simulink model "BWQWFPIDa"  (Simulink 8.3)
settings: Solver=ode45  SolverMode=SingleTasking  StartTime=0.0  StopTime=1000  FixedStep=20  RelTol=1e-3
settings Model: Creator=Zhu Supeng  LastModifiedBy=Zhu Supeng
settings DataIOCC: SignalLoggingName=sigsOut
settings DebuggingCC: SaveWithParameterizedLinksMsg=none  SignalResolutionControl=TryResolveAllWithWarning  SolverPrmCheckMsg=none  MultiTaskDSMMsg=warning  MultiTaskCondExecSysMsg=none  StateNameClashWarn=none
settings HardwareCC: TargetUnknown=on
settings RTWCC: IncludeERTFirstTime=on

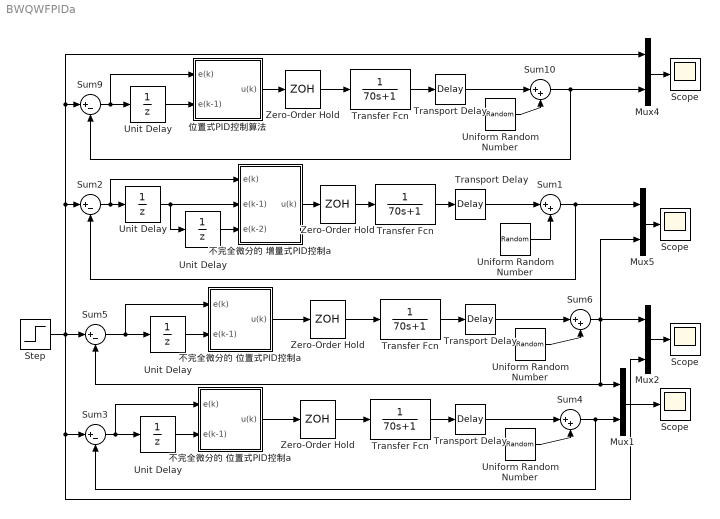
== system BWQWFPIDa ==
  "  Scope " : Scope
      settings: YMin=-3.5  YMax=1  SaveName=ScopeData3  MaxDataPoints=500000
  "  Transfer Fcn  " : TransferFcn  Denominator=[70 1]
  "  Transport Delay " : TransportDelay  DelayTime=80
  "  Unit Delay  " : UnitDelay  SampleTime=20
  " Scope " : Scope
      settings: YMin=-3.5  YMax=1  SaveName=BWQWFPIDary  MaxDataPoints=500000
  " Transfer Fcn " : TransferFcn  Denominator=[70 1]
  " Transport Delay " : TransportDelay  DelayTime=80
  " Unit Delay " : UnitDelay  SampleTime=20
  " Zero-Order Hold   " : ZeroOrderHold  SampleTime=20
  " 不完全微分的 位置式PID控制a " : Subsystem
  Mux1 : Mux  Inputs=2
  Mux2 : Mux  Inputs=3
  Mux4 : Mux  Inputs=2
  Mux5 : Mux  Inputs=2
  Scope : Scope
      settings: YMin=-3.5  YMax=1  MaxDataPoints=500000
  "Scope " : Scope
      settings: YMin=-3.5  YMax=1  MaxDataPoints=500000
  Step : Step  Time=0  SampleTime=0
  Sum{1,4,6,10} (4 alike) : Sum  Inputs=|++  SaturateOnIntegerOverflow=on
  Sum{2..3,5,9} (4 alike) : Sum  Inputs=|+-  SaturateOnIntegerOverflow=on
  Transfer Fcn : TransferFcn  Denominator=[70 1]
  "Transfer Fcn " : TransferFcn  Denominator=[70 1]
  Transport Delay : TransportDelay  DelayTime=80
  "Transport Delay " : TransportDelay  DelayTime=80
  Uniform Random Number : UniformRandomNumber  Minimum=-0.01  Maximum=0.01  SampleTime=20
  "Uniform Random Number " : UniformRandomNumber  Minimum=-0.01  Maximum=0.01  SampleTime=20
  "Uniform Random Number  " : UniformRandomNumber  Minimum=-0.01  Maximum=0.01  SampleTime=20
  "Uniform Random Number    " : UniformRandomNumber  Minimum=-0.01  Maximum=0.01  SampleTime=20
  Unit Delay : UnitDelay  SampleTime=20
  "Unit Delay " : UnitDelay  SampleTime=20
  "Unit Delay  " : UnitDelay  SampleTime=20
  Zero-Order Hold : ZeroOrderHold  SampleTime=20
  "Zero-Order Hold " : ZeroOrderHold  SampleTime=20
  "Zero-Order Hold  " : ZeroOrderHold  SampleTime=20
  不完全微分的 位置式PID控制a : Subsystem
  不完全微分的 增量式PID控制a : Subsystem
  "位置式PID控制算法 " : Subsystem
  wires:
  Step/1 -> Sum9/1, Mux4/1, Sum2/1, Sum5/1, Sum3/1, Mux2/3
  Transfer Fcn/1 -> Transport Delay/1
  "位置式PID控制算法 "/1(u(k)) -> Zero-Order Hold/1
  Unit Delay/1 -> "位置式PID控制算法 "/2(e(k-1))
  Sum9/1 -> Unit Delay/1, "位置式PID控制算法 "/1(e(k))
  Zero-Order Hold/1 -> Transfer Fcn/1
  Uniform Random Number/1 -> Sum10/2
  Transport Delay/1 -> Sum10/1
  Sum10/1 -> Sum9/2, Mux4/2
  Mux4/1 -> Scope/1
  "Transfer Fcn "/1 -> "Transport Delay "/1
  不完全微分的 增量式PID控制a/1(u(k)) -> "Zero-Order Hold "/1
  Sum2/1 -> "Unit Delay "/1, 不完全微分的 增量式PID控制a/1(e(k))
  Mux5/1 -> "Scope "/1
  "Transport Delay "/1 -> Sum1/1
  Sum1/1 -> Mux5/1, Sum2/2
  "Zero-Order Hold "/1 -> "Transfer Fcn "/1
  "Unit Delay "/1 -> "Unit Delay  "/1, 不完全微分的 增量式PID控制a/2(e(k-1))
  "Unit Delay  "/1 -> 不完全微分的 增量式PID控制a/3(e(k-2))
  " Transfer Fcn "/1 -> " Transport Delay "/1
  不完全微分的 位置式PID控制a/1(u(k)) -> "Zero-Order Hold  "/1
  " Unit Delay "/1 -> 不完全微分的 位置式PID控制a/2(e(k-1))
  Sum5/1 -> " Unit Delay "/1, 不完全微分的 位置式PID控制a/1(e(k))
  Mux2/1 -> " Scope "/1
  "Uniform Random Number  "/1 -> Sum6/2
  Sum6/1 -> Mux2/1, Mux5/2, Sum5/2, Mux1/1
  " Transport Delay "/1 -> Sum6/1
  "Zero-Order Hold  "/1 -> " Transfer Fcn "/1
  "Uniform Random Number "/1 -> Sum1/2
  "  Transfer Fcn  "/1 -> "  Transport Delay "/1
  " 不完全微分的 位置式PID控制a "/1(u(k)) -> " Zero-Order Hold   "/1
  "  Unit Delay  "/1 -> " 不完全微分的 位置式PID控制a "/2(e(k-1))
  Sum3/1 -> " 不完全微分的 位置式PID控制a "/1(e(k)), "  Unit Delay  "/1
  "Uniform Random Number    "/1 -> Sum4/2
  "  Transport Delay "/1 -> Sum4/1
  " Zero-Order Hold   "/1 -> "  Transfer Fcn  "/1
  Mux1/1 -> "  Scope "/1
  Sum4/1 -> Mux1/2, Sum3/2

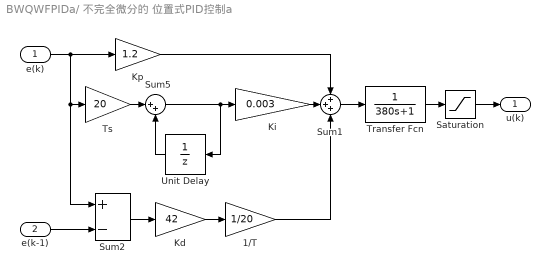
== system BWQWFPIDa/ 不完全微分的 位置式PID控制a  ==
  e(k) : Inport
  e(k-1) : Inport  Port=2
  1/T : Gain  Gain=1/20  SaturateOnIntegerOverflow=on  OutDataTypeStr=Inherit: Same as input  ParamDataTypeStr=Inherit: Same as input
  Kd : Gain  Gain=42  SaturateOnIntegerOverflow=on  OutDataTypeStr=Inherit: Same as input  ParamDataTypeStr=Inherit: Same as input
  Ki : Gain  Gain=0.003  SaturateOnIntegerOverflow=on  OutDataTypeStr=Inherit: Same as input  ParamDataTypeStr=Inherit: Same as input
  Kp : Gain  Gain=1.2  SaturateOnIntegerOverflow=on  OutDataTypeStr=Inherit: Same as input  ParamDataTypeStr=Inherit: Same as input
  Saturation : Saturate  UpperLimit=10  LowerLimit=-10
  Sum1 : Sum  Inputs=+++  SaturateOnIntegerOverflow=on
  Sum2 : Sum  Inputs=+-  SaturateOnIntegerOverflow=on
  Sum5 : Sum  Inputs=|++  SaturateOnIntegerOverflow=on
  Transfer Fcn : TransferFcn  Denominator=[380 1]
  Ts : Gain  Gain=20  SaturateOnIntegerOverflow=on  OutDataTypeStr=Inherit: Same as input  ParamDataTypeStr=Inherit: Same as input
  Unit Delay : UnitDelay  SampleTime=20
  u(k) : Outport
  wires:
  Ki/1 -> Sum1/2
  1/T/1 -> Sum1/3
  Sum2/1 -> Kd/1
  e(k)/1 -> Kp/1, Ts/1, Sum2/1
  Kp/1 -> Sum1/1
  e(k-1)/1 -> Sum2/2
  Kd/1 -> 1/T/1
  Ts/1 -> Sum5/1
  Sum5/1 -> Unit Delay/1, Ki/1
  Unit Delay/1 -> Sum5/2
  Sum1/1 -> Transfer Fcn/1
  Saturation/1 -> u(k)/1
  Transfer Fcn/1 -> Saturation/1

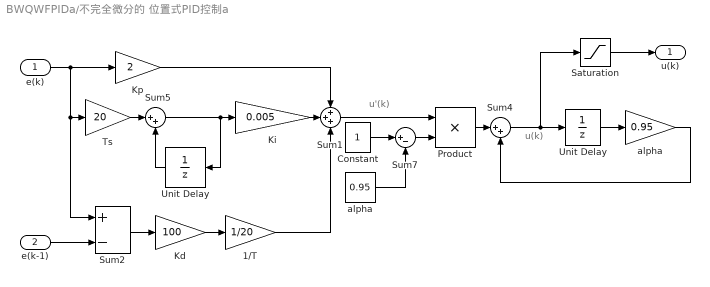
== system BWQWFPIDa/不完全微分的 位置式PID控制a ==
  note: u'(k)
  note: u(k)
  e(k) : Inport
  e(k-1) : Inport  Port=2
  1/T : Gain  Gain=1/20  SaturateOnIntegerOverflow=on  OutDataTypeStr=Inherit: Same as input  ParamDataTypeStr=Inherit: Same as input
  Constant : Constant
  Kd : Gain  Gain=100  SaturateOnIntegerOverflow=on  OutDataTypeStr=Inherit: Same as input  ParamDataTypeStr=Inherit: Same as input
  Ki : Gain  Gain=0.005  SaturateOnIntegerOverflow=on  OutDataTypeStr=Inherit: Same as input  ParamDataTypeStr=Inherit: Same as input
  Kp : Gain  Gain=2  SaturateOnIntegerOverflow=on  OutDataTypeStr=Inherit: Same as input  ParamDataTypeStr=Inherit: Same as input
  Product : Product  SaturateOnIntegerOverflow=on  OutDataTypeStr=Inherit: Same as first input
  Saturation : Saturate  UpperLimit=10  LowerLimit=-10
  Sum1 : Sum  Inputs=+++  SaturateOnIntegerOverflow=on
  Sum2 : Sum  Inputs=+-  SaturateOnIntegerOverflow=on
  Sum4 : Sum  Inputs=|++  SaturateOnIntegerOverflow=on
  Sum5 : Sum  Inputs=|++  SaturateOnIntegerOverflow=on
  Sum7 : Sum  Inputs=|+-  SaturateOnIntegerOverflow=on
  Ts : Gain  Gain=20  SaturateOnIntegerOverflow=on  OutDataTypeStr=Inherit: Same as input  ParamDataTypeStr=Inherit: Same as input
  Unit Delay : UnitDelay  SampleTime=20
  "Unit Delay " : UnitDelay  SampleTime=20
  alpha : Constant  Value=0.95
  "alpha " : Gain  Gain=0.95  SaturateOnIntegerOverflow=on  OutDataTypeStr=Inherit: Same as input  ParamDataTypeStr=Inherit: Same as input
  u(k) : Outport
  wires:
  "alpha "/1 -> Sum4/2
  "Unit Delay "/1 -> "alpha "/1
  Sum4/1 -> Saturation/1, "Unit Delay "/1
  Unit Delay/1 -> Sum5/2
  Sum5/1 -> Ki/1, Unit Delay/1
  Ts/1 -> Sum5/1
  Kd/1 -> 1/T/1
  e(k-1)/1 -> Sum2/2
  Saturation/1 -> u(k)/1
  Kp/1 -> Sum1/1
  e(k)/1 -> Sum2/1, Ts/1, Kp/1
  alpha/1 -> Sum7/2
  Constant/1 -> Sum7/1
  Sum2/1 -> Kd/1
  Product/1 -> Sum4/1
  Sum1/1 -> Product/1
  1/T/1 -> Sum1/3
  Ki/1 -> Sum1/2
  Sum7/1 -> Product/2

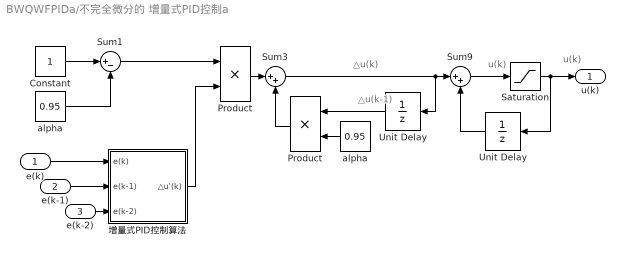
== system BWQWFPIDa/不完全微分的 增量式PID控制a ==
  note: △u(k)
  note: u(k)
  note: u(k)
  note: △u(k-1)
  e(k) : Inport
  e(k-1) : Inport  Port=2
  e(k-2) : Inport  Port=3
  Constant : Constant
  Product : Product  SaturateOnIntegerOverflow=on  OutDataTypeStr=Inherit: Same as first input
  "Product " : Product  SaturateOnIntegerOverflow=on  OutDataTypeStr=Inherit: Same as first input
  "Saturation " : Saturate  UpperLimit=10  LowerLimit=-10
  Sum1 : Sum  Inputs=|+-  SaturateOnIntegerOverflow=on
  Sum3 : Sum  Inputs=|++  SaturateOnIntegerOverflow=on
  Sum9 : Sum  Inputs=|++  SaturateOnIntegerOverflow=on
  Unit Delay : UnitDelay  SampleTime=20
  "Unit Delay " : UnitDelay  SampleTime=20
  alpha : Constant  Value=0.95
  "alpha " : Constant  Value=0.95
  增量式PID控制算法 : Subsystem
  u(k) : Outport
  wires:
  Sum3/1 -> Sum9/1, "Unit Delay "/1
  Sum9/1 -> "Saturation "/1
  "Saturation "/1 -> Unit Delay/1, u(k)/1
  Unit Delay/1 -> Sum9/2
  Constant/1 -> Sum1/1
  "alpha "/1 -> Sum1/2
  Sum1/1 -> "Product "/1
  增量式PID控制算法/1("△u'(k) ") -> "Product "/2
  "Unit Delay "/1 -> Product/1
  alpha/1 -> Product/2
  Product/1 -> Sum3/2
  "Product "/1 -> Sum3/1
  e(k)/1 -> 增量式PID控制算法/1(e(k))
  e(k-1)/1 -> 增量式PID控制算法/2(e(k-1))
  e(k-2)/1 -> 增量式PID控制算法/3(e(k-2))

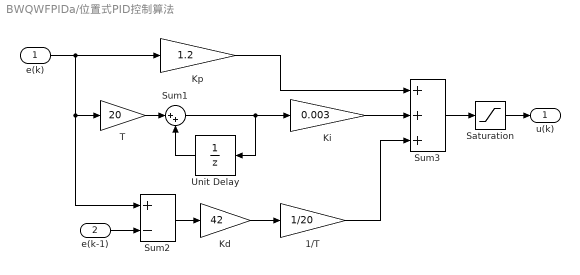
== system BWQWFPIDa/位置式PID控制算法  ==
  e(k) : Inport
  e(k-1) : Inport  Port=2
  1/T : Gain  Gain=1/20  SaturateOnIntegerOverflow=on  OutDataTypeStr=Inherit: Same as input  ParamDataTypeStr=Inherit: Same as input
  Kd : Gain  Gain=42  SaturateOnIntegerOverflow=on  OutDataTypeStr=Inherit: Same as input  ParamDataTypeStr=Inherit: Same as input
  Ki : Gain  Gain=0.003  SaturateOnIntegerOverflow=on  OutDataTypeStr=Inherit: Same as input  ParamDataTypeStr=Inherit: Same as input
  Kp : Gain  Gain=1.2  SaturateOnIntegerOverflow=on  OutDataTypeStr=Inherit: Same as input  ParamDataTypeStr=Inherit: Same as input
  Saturation : Saturate  UpperLimit=10  LowerLimit=-10
  Sum1 : Sum  Inputs=|++  SaturateOnIntegerOverflow=on
  Sum2 : Sum  Inputs=+-  SaturateOnIntegerOverflow=on
  Sum3 : Sum  Inputs=+++  SaturateOnIntegerOverflow=on
  T : Gain  Gain=20  SaturateOnIntegerOverflow=on  OutDataTypeStr=Inherit: Same as input  ParamDataTypeStr=Inherit: Same as input
  "Unit Delay " : UnitDelay  SampleTime=20
  u(k) : Outport
  wires:
  Sum2/1 -> Kd/1
  e(k)/1 -> Kp/1, Sum2/1, T/1
  Kp/1 -> Sum3/1
  Ki/1 -> Sum3/2
  Sum3/1 -> Saturation/1
  Saturation/1 -> u(k)/1
  Kd/1 -> 1/T/1
  e(k-1)/1 -> Sum2/2
  1/T/1 -> Sum3/3
  Sum1/1 -> "Unit Delay "/1, Ki/1
  "Unit Delay "/1 -> Sum1/2
  T/1 -> Sum1/1

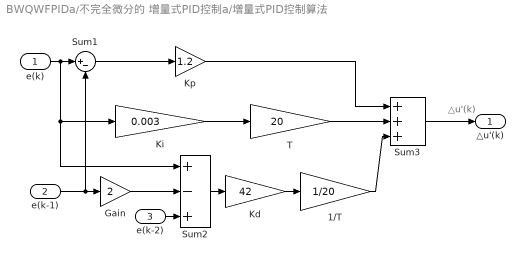
== system BWQWFPIDa/不完全微分的 增量式PID控制a/增量式PID控制算法 ==
  note: △u'(k)
  e(k) : Inport
  e(k-1) : Inport  Port=2
  e(k-2) : Inport  Port=3
  1/T : Gain  Gain=1/20  SaturateOnIntegerOverflow=on  OutDataTypeStr=Inherit: Same as input  ParamDataTypeStr=Inherit: Same as input
  Gain : Gain  Gain=2  SaturateOnIntegerOverflow=on  OutDataTypeStr=Inherit: Same as input  ParamDataTypeStr=Inherit: Same as input
  Kd : Gain  Gain=42  SaturateOnIntegerOverflow=on  OutDataTypeStr=Inherit: Same as input  ParamDataTypeStr=Inherit: Same as input
  Ki : Gain  Gain=0.003  SaturateOnIntegerOverflow=on  OutDataTypeStr=Inherit: Same as input  ParamDataTypeStr=Inherit: Same as input
  Kp : Gain  Gain=1.2  SaturateOnIntegerOverflow=on  OutDataTypeStr=Inherit: Same as input  ParamDataTypeStr=Inherit: Same as input
  Sum1 : Sum  Inputs=|+-  SaturateOnIntegerOverflow=on
  Sum2 : Sum  Inputs=+-+  SaturateOnIntegerOverflow=on
  Sum3 : Sum  Inputs=+++  SaturateOnIntegerOverflow=on
  T : Gain  Gain=20  SaturateOnIntegerOverflow=on  OutDataTypeStr=Inherit: Same as input  ParamDataTypeStr=Inherit: Same as input
  "△u'(k) " : Outport
  wires:
  Sum1/1 -> Kp/1
  Gain/1 -> Sum2/2
  Sum2/1 -> Kd/1
  e(k-1)/1 -> Gain/1, Sum1/2
  e(k-2)/1 -> Sum2/3
  e(k)/1 -> Sum1/1, Sum2/1, Ki/1
  Kp/1 -> Sum3/1
  Ki/1 -> T/1
  Sum3/1 -> "△u'(k) "/1
  Kd/1 -> 1/T/1
  T/1 -> Sum3/2
  1/T/1 -> Sum3/3
